simulink model "extkalmfilt_simQ4"  (R2020b)
settings: Solver=VariableStepAuto  StartTime=0.0  StopTime=tf  RelTol=1e-3
model workspace (MATLAB code in the model file):
  | %global Cv Ac Ts Fi_ss Qtrue
  | 
  | % Tank properties
  | Cv1 = 0.8;Cv2=0.8;
  | A1=1.2;A2=1.2;
  | 
  | % Steady-state flow
  | Fi_ss = 2;
  | 
  | % Initial conditions
  | h1_ss = (Fi_ss/Cv1)^2;
  | h2_ss = (Cv1/Cv2)^2*h1_ss;
  | x0 =[h1_ss;h2_ss];
  | 
  | % Sampling interval
  | Ts = 0.1;
  | 
  | % Final time and time vector
  | tf = 127.4;
  | kvec = (0:Ts:tf)';
  | N = length(kvec);
  | 
  | % Input sequence (deviation from steady-state)
  | ukvec = idinput(N,'prbs',[0 0.2],[-1 1]);
  | simin = [kvec ukvec];
  | 
  | % Process and measurement noise covariances
  | Qtrue = diag([0.2,0.1]);
  | Rtrue = 0.1;
libraries: sharedTrackingLibrary x1
settings Model: OrderedModelArguments=off  Creator=arun  LastModifiedBy=HP

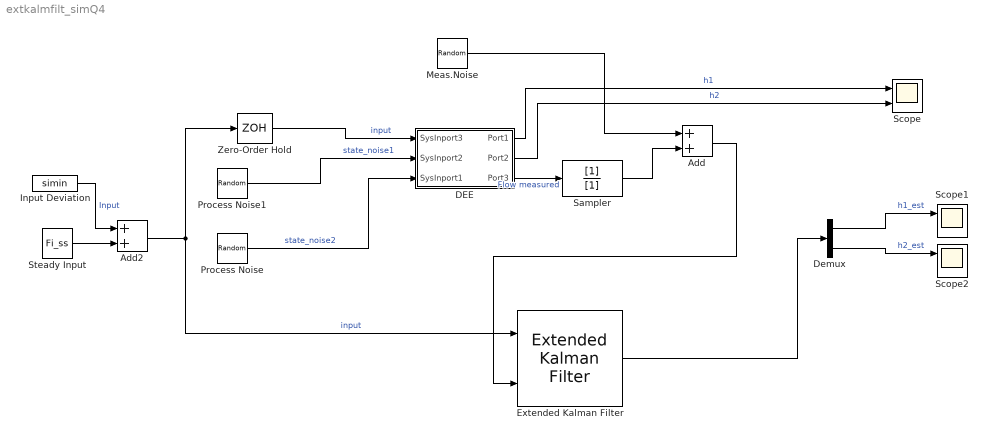
== system extkalmfilt_simQ4 ==
  Add : Sum
  Add2 : Sum
  DEE : Subsystem  mask(Differential Equation Editor (DEE)){}
      settings: OpenFcn=diffeqed
      mask Display: disp('Liquid Level \n System')
  Demux : Demux  Outputs=2
  Extended Kalman Filter : sharedTrackingLibrary/Extended Kalman Filter  StateTransitionFcn=liqlstatetrans_fun  HasStateTransitionJacobianFcn=off  HasAdditiveProcessNoise=Additive  ProcessNoise=Qtrue  HasTimeVaryingProcessNoise=off  HasStateTransitionFcnExtraArgument=1  InitialState=[h1_ss;h2_ss]  InitialStateCovariance=0.1  MeasurementFcn1=liqlmeas_fun  HasMeasurementJacobianFcn1=off  HasMeasurementEnablePort1=off  HasAdditiveMeasurementNoise1=Additive  MeasurementNoise1=Rtrue  HasTimeVaryingMeasurementNoise1=off  HasMeasurementFcnExtraArgument1=0  MeasurementFcn2=myMeasurementFcn  HasMeasurementJacobianFcn2=off  HasMeasurementEnablePort2=off  HasAdditiveMeasurementNoise2=Additive  MeasurementNoise2=1  HasTimeVaryingMeasurementNoise2=off  HasMeasurementFcnExtraArgument2=0  MeasurementFcn3=myMeasurementFcn  HasMeasurementJacobianFcn3=off  HasMeasurementEnablePort3=off  HasAdditiveMeasurementNoise3=Additive  MeasurementNoise3=1  HasTimeVaryingMeasurementNoise3=off  HasMeasurementFcnExtraArgument3=0  MeasurementFcn4=myMeasurementFcn  HasMeasurementJacobianFcn4=off  HasMeasurementEnablePort4=off  HasAdditiveMeasurementNoise4=Additive  MeasurementNoise4=1  HasTimeVaryingMeasurementNoise4=off  HasMeasurementFcnExtraArgument4=0  MeasurementFcn5=myMeasurementFcn  HasMeasurementJacobianFcn5=off  HasMeasurementEnablePort5=off  HasAdditiveMeasurementNoise5=Additive  MeasurementNoise5=1  HasTimeVaryingMeasurementNoise5=off  HasMeasurementFcnExtraArgument5=0  EnableMultirate=off  StateTransitionFcnSampleTime=1  MeasurementFcn1SampleTime=1  MeasurementFcn2SampleTime=1  MeasurementFcn3SampleTime=1  MeasurementFcn4SampleTime=1  MeasurementFcn5SampleTime=1  UseCurrentEstimator=on  OutputStateCovariance=off  DataType=double  SampleTime=Ts  NumberOfMeasurements=1
      settings: SourceProductBaseCode=CT,DR,TF,ID,LP,NV,AR,RO,RR,UV,VE
  Input Deviation : FromWorkspace  VariableName=simin  SampleTime=Ts  Interpolate=off  OutputAfterFinalValue=Holding final value
  Meas.Noise : RandomNumber  Variance=Rtrue  Seed=4781  SampleTime=Ts
  Process Noise : RandomNumber  Variance=Qtrue(2,2)  Seed=38760  SampleTime=Ts
  Process Noise1 : RandomNumber  Variance=Qtrue(1)  Seed=1234  SampleTime=Ts
  Sampler : DiscreteFilter  Denominator=[1]  SampleTime=Ts
  Scope : Scope  NumInputPorts=2
  Scope1 : Scope  NumInputPorts=2
  Scope2 : Scope  NumInputPorts=2
  Steady Input : Constant  Value=Fi_ss  SampleTime=Ts
  Zero-Order Hold : ZeroOrderHold  SampleTime=Ts
  wires:
  Meas.Noise/1 -> Add/1
  Add/1 -> Extended Kalman Filter/2
  Extended Kalman Filter/1 -> Demux/1
  Steady Input/1 -> Add2/2
  Add2/1 -> Extended Kalman Filter/1, Zero-Order Hold/1  "input"
  Input Deviation/1 -> Add2/1  "Input"
  Sampler/1 -> Add/2
  Process Noise1/1 -> DEE/2(SysInport2)  "state_noise1"
  Process Noise/1 -> DEE/3(SysInport1)  "state_noise2"
  Zero-Order Hold/1 -> DEE/1(SysInport3)  "input"
  DEE/3(Port3) -> Sampler/1  "Flow measured"
  DEE/2(Port2) -> Scope/2  "h2"
  DEE/1(Port1) -> Scope/1  "h1"
  Demux/1 -> Scope1/1  "h1_est"
  Demux/2 -> Scope2/1  "h2_est"

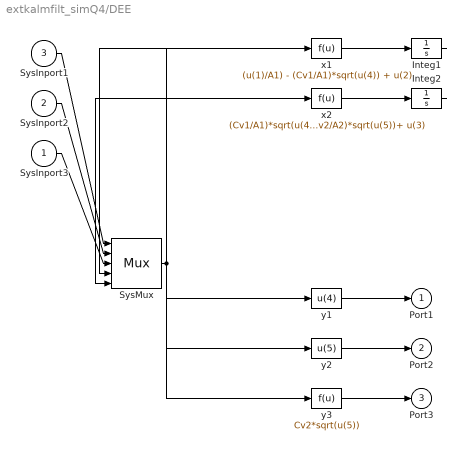
== system extkalmfilt_simQ4/DEE ==
  SysInport3 : Inport
  SysInport2 : Inport  Port=2
  SysInport1 : Inport  Port=3
  Integ1 : Integrator  InitialCondition=x0(1)
  Integ2 : Integrator  InitialCondition=x0(2)
  SysMux : Mux  Inputs=5
  x1 : Fcn  Expr=(u(1)/A1) - (Cv1/A1)*sqrt(u(4)) + u(2)
  x2 : Fcn  Expr=(Cv1/A1)*sqrt(u(4)) - (Cv2/A2)*sqrt(u(5))+ u(3)
  y1 : Fcn  Expr=u(4)
  y2 : Fcn  Expr=u(5)
  y3 : Fcn  Expr=Cv2*sqrt(u(5))
  Port1 : Outport
  Port2 : Outport  Port=2
  Port3 : Outport  Port=3
  wires:
  SysInport1/1 -> SysMux/1
  SysInport2/1 -> SysMux/2
  SysInport3/1 -> SysMux/3
  SysMux/1 -> x1/1, x2/1, y1/1, y2/1, y3/1
  x1/1 -> Integ1/1
  Integ1/1 -> SysMux/4
  x2/1 -> Integ2/1
  Integ2/1 -> SysMux/5
  y1/1 -> Port1/1
  y2/1 -> Port2/1
  y3/1 -> Port3/1
